simulink model "v_0"  (R2017a)
settings: Solver=FixedStepDiscrete  StartTime=0.0  StopTime=5  FixedStep=0.01  RelTol=1e-3
libraries: simulink x1
settings Model: Creator=Vasilii  LastModifiedBy=Vasilii

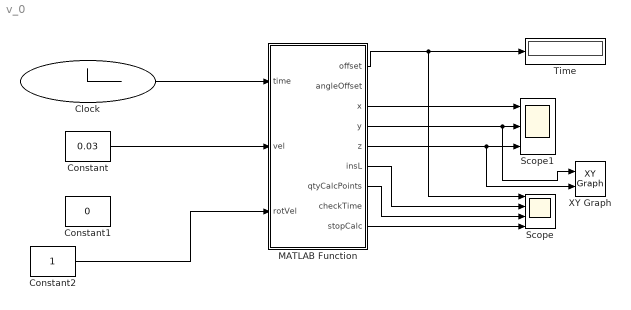
== system v_0 ==
  Clock : Clock
  Constant : Constant  Value=0.03
  Constant1 : Constant  Value=0
  Constant2 : Constant
  MATLAB Function : MATLAB Function  TreatAsAtomicUnit=on
  Scope : Scope  NumInputPorts=4
  Scope1 : Scope  NumInputPorts=3
  Time : Display
      settings: Decimation=4
  XY Graph : simulink/Sinks/XY Graph  xmin=-4  xmax=4  ymin=-4  ymax=4  st=-1
  wires:
  Constant/1 -> MATLAB Function/2(vel)
  Clock/1 -> MATLAB Function/1(time)
  MATLAB Function/1(offset) -> Scope/1, Time/1
  MATLAB Function/9(stopCalc) -> Scope/4
  MATLAB Function/7(qtyCalcPoints) -> Scope/3
  MATLAB Function/6(insL) -> Scope/2
  MATLAB Function/3(x) -> Scope1/1
  MATLAB Function/4(y) -> XY Graph/1, Scope1/2
  MATLAB Function/5(z) -> XY Graph/2, Scope1/3
  Constant2/1 -> MATLAB Function/3(rotVel)

== matlab function v_0/MATLAB Function ==
  data: time input; offset output; vel input; angleOffset output; x output; y output; z output; insL output; qtyCalcPoints output; checkTime output; stopCalc output; rotVel input
function [offset,angleOffset,x,y,z,insL,qtyCalcPoints,checkTime,stopCalc] = fcn(time,vel,rotVel)

[offset,angleOffset,x,y,z,insL,qtyCalcPoints,checkTime,stopCalc] = CalcFunction_v_0(time,vel,rotVel);
